simulink model "GalacticSoupLogical"  (R2025b)
settings: Solver=VariableStepAuto  StartTime=0.0  StopTime=10.0  RelTol=1e-3
settings Model: DataDictionary=GalacticSoupLogicalInterfaces.sldd  Creator=sarah  LastModifiedBy=sarah

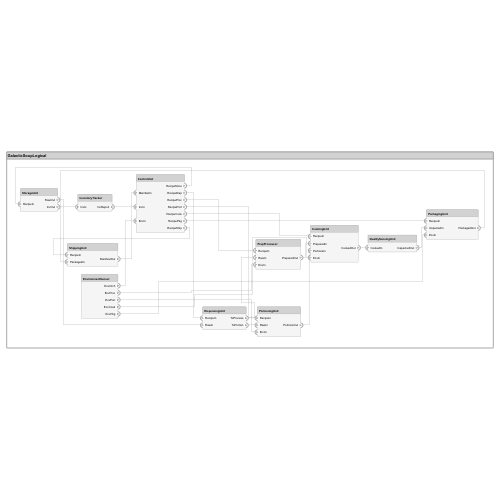
[thumbnail: Simulink's stored preview of the top-level diagram]
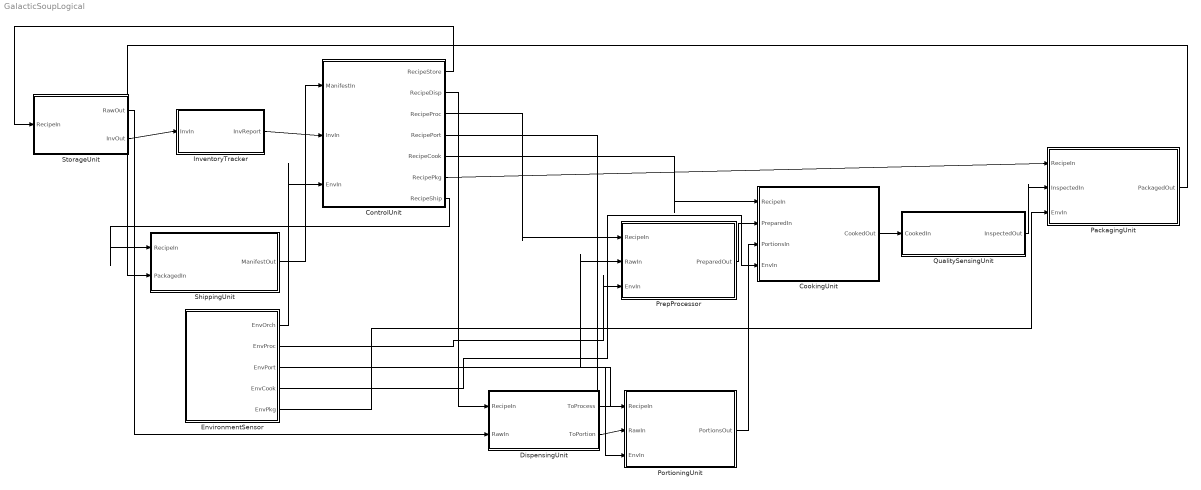
== system GalacticSoupLogical ==
  ControlUnit : Subsystem
      settings: PortSchema="{\"entries\":[{\"content\":{\"headerSize\":26,\"margin\":15,\"minimumSpacing\":25,\"sides\":[{\"content\":{\"connectorIds\":[\"In1\",\"In2\",\"In3\"]},\"type\":\"ConnectorPlacement.EquallySpacedRectSide\",\"uuid\":\"e444b18e-2ceb-4425-8803-e6c31b1fcd82\"},{\"content\":{\"connectorIds\":[\"Out1\",\"Out2\",\"Out3\",\"Out4\",\"Out5\",\"Out6\",\"Out7\"],\"side\":\"RIGHT\"},\"type\":\"ConnectorPlacement.EquallySpacedRectSide\",\"uuid\":\"f4aec6c9-b52d-4884-9c27-2bb07598a416\"},{\"content\":{\"side\":\"TOP\"},\"type\":\"ConnectorPlacement.EquallySpacedRectSide\",\"uuid\":\"1037694d-1bab-41f9-830b-c4a2d0bddcad\"}]},\"type\":\"ConnectorPlacement.EquallySpacedConnector\",\"uuid\":\"fcfa453c-694a-4044-b0a2-73b33e092223\"}],\"packageUris\":[\"http://schema.mathworks.com/mf0/Connector/R2020b\"],\"version\":\"1.0\"}"
  CookingUnit : Subsystem
      settings: PortSchema="{\"entries\":[{\"content\":{\"headerSize\":26,\"margin\":15,\"minimumSpacing\":25,\"sides\":[{\"content\":{\"connectorIds\":[\"In1\",\"In2\",\"In3\",\"In4\"]},\"type\":\"ConnectorPlacement.EquallySpacedRectSide\",\"uuid\":\"e444b18e-2ceb-4425-8803-e6c31b1fcd82\"},{\"content\":{\"connectorIds\":[\"Out1\"],\"side\":\"RIGHT\"},\"type\":\"ConnectorPlacement.EquallySpacedRectSide\",\"uuid\":\"f4aec6c9-b52d-4884-9c27-2bb07598a416\"},{\"content\":{\"side\":\"TOP\"},\"type\":\"ConnectorPlacement.EquallySpacedRectSide\",\"uuid\":\"1037694d-1bab-41f9-830b-c4a2d0bddcad\"}]},\"type\":\"ConnectorPlacement.EquallySpacedConnector\",\"uuid\":\"fcfa453c-694a-4044-b0a2-73b33e092223\"}],\"packageUris\":[\"http://schema.mathworks.com/mf0/Connector/R2020b\"],\"version\":\"1.0\"}"
  DispensingUnit : Subsystem
      settings: PortSchema="{\"entries\":[{\"content\":{\"headerSize\":26,\"margin\":15,\"minimumSpacing\":25,\"sides\":[{\"content\":{\"connectorIds\":[\"In1\",\"In2\"]},\"type\":\"ConnectorPlacement.EquallySpacedRectSide\",\"uuid\":\"e444b18e-2ceb-4425-8803-e6c31b1fcd82\"},{\"content\":{\"connectorIds\":[\"Out1\",\"Out2\"],\"side\":\"RIGHT\"},\"type\":\"ConnectorPlacement.EquallySpacedRectSide\",\"uuid\":\"f4aec6c9-b52d-4884-9c27-2bb07598a416\"},{\"content\":{\"side\":\"TOP\"},\"type\":\"ConnectorPlacement.EquallySpacedRectSide\",\"uuid\":\"1037694d-1bab-41f9-830b-c4a2d0bddcad\"}]},\"type\":\"ConnectorPlacement.EquallySpacedConnector\",\"uuid\":\"fcfa453c-694a-4044-b0a2-73b33e092223\"}],\"packageUris\":[\"http://schema.mathworks.com/mf0/Connector/R2020b\"],\"version\":\"1.0\"}"
  EnvironmentSensor : Subsystem
      settings: PortSchema="{\"entries\":[{\"content\":{\"headerSize\":26,\"margin\":15,\"minimumSpacing\":25,\"sides\":[{\"content\":{},\"type\":\"ConnectorPlacement.EquallySpacedRectSide\",\"uuid\":\"e444b18e-2ceb-4425-8803-e6c31b1fcd82\"},{\"content\":{\"connectorIds\":[\"Out1\",\"Out2\",\"Out3\",\"Out4\",\"Out5\"],\"side\":\"RIGHT\"},\"type\":\"ConnectorPlacement.EquallySpacedRectSide\",\"uuid\":\"f4aec6c9-b52d-4884-9c27-2bb07598a416\"},{\"content\":{\"side\":\"TOP\"},\"type\":\"ConnectorPlacement.EquallySpacedRectSide\",\"uuid\":\"1037694d-1bab-41f9-830b-c4a2d0bddcad\"}]},\"type\":\"ConnectorPlacement.EquallySpacedConnector\",\"uuid\":\"fcfa453c-694a-4044-b0a2-73b33e092223\"}],\"packageUris\":[\"http://schema.mathworks.com/mf0/Connector/R2020b\"],\"version\":\"1.0\"}"
  InventoryTracker : Subsystem
      settings: PortSchema="{\"entries\":[{\"content\":{\"headerSize\":26,\"margin\":15,\"minimumSpacing\":25,\"sides\":[{\"content\":{\"connectorIds\":[\"In1\"]},\"type\":\"ConnectorPlacement.EquallySpacedRectSide\",\"uuid\":\"e444b18e-2ceb-4425-8803-e6c31b1fcd82\"},{\"content\":{\"connectorIds\":[\"Out1\"],\"side\":\"RIGHT\"},\"type\":\"ConnectorPlacement.EquallySpacedRectSide\",\"uuid\":\"f4aec6c9-b52d-4884-9c27-2bb07598a416\"},{\"content\":{\"side\":\"TOP\"},\"type\":\"ConnectorPlacement.EquallySpacedRectSide\",\"uuid\":\"1037694d-1bab-41f9-830b-c4a2d0bddcad\"}]},\"type\":\"ConnectorPlacement.EquallySpacedConnector\",\"uuid\":\"fcfa453c-694a-4044-b0a2-73b33e092223\"}],\"packageUris\":[\"http://schema.mathworks.com/mf0/Connector/R2020b\"],\"version\":\"1.0\"}"
  PackagingUnit : Subsystem
      settings: PortSchema="{\"entries\":[{\"content\":{\"headerSize\":26,\"margin\":15,\"minimumSpacing\":25,\"sides\":[{\"content\":{\"connectorIds\":[\"In1\",\"In2\",\"In3\"]},\"type\":\"ConnectorPlacement.EquallySpacedRectSide\",\"uuid\":\"e444b18e-2ceb-4425-8803-e6c31b1fcd82\"},{\"content\":{\"connectorIds\":[\"Out1\"],\"side\":\"RIGHT\"},\"type\":\"ConnectorPlacement.EquallySpacedRectSide\",\"uuid\":\"f4aec6c9-b52d-4884-9c27-2bb07598a416\"},{\"content\":{\"side\":\"TOP\"},\"type\":\"ConnectorPlacement.EquallySpacedRectSide\",\"uuid\":\"1037694d-1bab-41f9-830b-c4a2d0bddcad\"}]},\"type\":\"ConnectorPlacement.EquallySpacedConnector\",\"uuid\":\"fcfa453c-694a-4044-b0a2-73b33e092223\"}],\"packageUris\":[\"http://schema.mathworks.com/mf0/Connector/R2020b\"],\"version\":\"1.0\"}"
  PortioningUnit : Subsystem
      settings: PortSchema="{\"entries\":[{\"content\":{\"headerSize\":26,\"margin\":15,\"minimumSpacing\":25,\"sides\":[{\"content\":{\"connectorIds\":[\"In1\",\"In2\",\"In3\"]},\"type\":\"ConnectorPlacement.EquallySpacedRectSide\",\"uuid\":\"e444b18e-2ceb-4425-8803-e6c31b1fcd82\"},{\"content\":{\"connectorIds\":[\"Out1\"],\"side\":\"RIGHT\"},\"type\":\"ConnectorPlacement.EquallySpacedRectSide\",\"uuid\":\"f4aec6c9-b52d-4884-9c27-2bb07598a416\"},{\"content\":{\"side\":\"TOP\"},\"type\":\"ConnectorPlacement.EquallySpacedRectSide\",\"uuid\":\"1037694d-1bab-41f9-830b-c4a2d0bddcad\"}]},\"type\":\"ConnectorPlacement.EquallySpacedConnector\",\"uuid\":\"fcfa453c-694a-4044-b0a2-73b33e092223\"}],\"packageUris\":[\"http://schema.mathworks.com/mf0/Connector/R2020b\"],\"version\":\"1.0\"}"
  PrepProcessor : Subsystem
      settings: PortSchema="{\"entries\":[{\"content\":{\"headerSize\":26,\"margin\":15,\"minimumSpacing\":25,\"sides\":[{\"content\":{\"connectorIds\":[\"In1\",\"In2\",\"In3\"]},\"type\":\"ConnectorPlacement.EquallySpacedRectSide\",\"uuid\":\"e444b18e-2ceb-4425-8803-e6c31b1fcd82\"},{\"content\":{\"connectorIds\":[\"Out1\"],\"side\":\"RIGHT\"},\"type\":\"ConnectorPlacement.EquallySpacedRectSide\",\"uuid\":\"f4aec6c9-b52d-4884-9c27-2bb07598a416\"},{\"content\":{\"side\":\"TOP\"},\"type\":\"ConnectorPlacement.EquallySpacedRectSide\",\"uuid\":\"1037694d-1bab-41f9-830b-c4a2d0bddcad\"}]},\"type\":\"ConnectorPlacement.EquallySpacedConnector\",\"uuid\":\"fcfa453c-694a-4044-b0a2-73b33e092223\"}],\"packageUris\":[\"http://schema.mathworks.com/mf0/Connector/R2020b\"],\"version\":\"1.0\"}"
  QualitySensingUnit : Subsystem
      settings: PortSchema="{\"entries\":[{\"content\":{\"headerSize\":26,\"margin\":15,\"minimumSpacing\":25,\"sides\":[{\"content\":{\"connectorIds\":[\"In1\"]},\"type\":\"ConnectorPlacement.EquallySpacedRectSide\",\"uuid\":\"e444b18e-2ceb-4425-8803-e6c31b1fcd82\"},{\"content\":{\"connectorIds\":[\"Out1\"],\"side\":\"RIGHT\"},\"type\":\"ConnectorPlacement.EquallySpacedRectSide\",\"uuid\":\"f4aec6c9-b52d-4884-9c27-2bb07598a416\"},{\"content\":{\"side\":\"TOP\"},\"type\":\"ConnectorPlacement.EquallySpacedRectSide\",\"uuid\":\"1037694d-1bab-41f9-830b-c4a2d0bddcad\"}]},\"type\":\"ConnectorPlacement.EquallySpacedConnector\",\"uuid\":\"fcfa453c-694a-4044-b0a2-73b33e092223\"}],\"packageUris\":[\"http://schema.mathworks.com/mf0/Connector/R2020b\"],\"version\":\"1.0\"}"
  ShippingUnit : Subsystem
      settings: PortSchema="{\"entries\":[{\"content\":{\"headerSize\":26,\"margin\":15,\"minimumSpacing\":25,\"sides\":[{\"content\":{\"connectorIds\":[\"In1\",\"In2\"]},\"type\":\"ConnectorPlacement.EquallySpacedRectSide\",\"uuid\":\"e444b18e-2ceb-4425-8803-e6c31b1fcd82\"},{\"content\":{\"connectorIds\":[\"Out1\"],\"side\":\"RIGHT\"},\"type\":\"ConnectorPlacement.EquallySpacedRectSide\",\"uuid\":\"f4aec6c9-b52d-4884-9c27-2bb07598a416\"},{\"content\":{\"side\":\"TOP\"},\"type\":\"ConnectorPlacement.EquallySpacedRectSide\",\"uuid\":\"1037694d-1bab-41f9-830b-c4a2d0bddcad\"}]},\"type\":\"ConnectorPlacement.EquallySpacedConnector\",\"uuid\":\"fcfa453c-694a-4044-b0a2-73b33e092223\"}],\"packageUris\":[\"http://schema.mathworks.com/mf0/Connector/R2020b\"],\"version\":\"1.0\"}"
  StorageUnit : Subsystem
      settings: PortSchema="{\"entries\":[{\"content\":{\"headerSize\":26,\"margin\":15,\"minimumSpacing\":25,\"sides\":[{\"content\":{\"connectorIds\":[\"In1\"]},\"type\":\"ConnectorPlacement.EquallySpacedRectSide\",\"uuid\":\"e444b18e-2ceb-4425-8803-e6c31b1fcd82\"},{\"content\":{\"connectorIds\":[\"Out1\",\"Out2\"],\"side\":\"RIGHT\"},\"type\":\"ConnectorPlacement.EquallySpacedRectSide\",\"uuid\":\"f4aec6c9-b52d-4884-9c27-2bb07598a416\"},{\"content\":{\"side\":\"TOP\"},\"type\":\"ConnectorPlacement.EquallySpacedRectSide\",\"uuid\":\"1037694d-1bab-41f9-830b-c4a2d0bddcad\"}]},\"type\":\"ConnectorPlacement.EquallySpacedConnector\",\"uuid\":\"fcfa453c-694a-4044-b0a2-73b33e092223\"}],\"packageUris\":[\"http://schema.mathworks.com/mf0/Connector/R2020b\"],\"version\":\"1.0\"}"
  wires:
  ShippingUnit/1(ManifestOut) -> ControlUnit/1(ManifestIn)
  StorageUnit/1(RawOut) -> DispensingUnit/2(RawIn)
  InventoryTracker/1(InvReport) -> ControlUnit/2(InvIn)
  StorageUnit/2(InvOut) -> InventoryTracker/1(InvIn)
  EnvironmentSensor/2(EnvProc) -> PrepProcessor/3(EnvIn)
  EnvironmentSensor/1(EnvOrch) -> ControlUnit/3(EnvIn)
  EnvironmentSensor/4(EnvCook) -> CookingUnit/4(EnvIn)
  EnvironmentSensor/3(EnvPort) -> PortioningUnit/3(EnvIn)
  EnvironmentSensor/5(EnvPkg) -> PackagingUnit/3(EnvIn)
  ControlUnit/1(RecipeStore) -> StorageUnit/1(RecipeIn)
  PrepProcessor/1(PreparedOut) -> CookingUnit/2(PreparedIn)
  ControlUnit/2(RecipeDisp) -> DispensingUnit/1(RecipeIn)
  ControlUnit/3(RecipeProc) -> PrepProcessor/1(RecipeIn)
  ControlUnit/4(RecipePort) -> PortioningUnit/1(RecipeIn)
  ControlUnit/5(RecipeCook) -> CookingUnit/1(RecipeIn)
  ControlUnit/6(RecipePkg) -> PackagingUnit/1(RecipeIn)
  ControlUnit/7(RecipeShip) -> ShippingUnit/1(RecipeIn)
  DispensingUnit/1(ToProcess) -> PrepProcessor/2(RawIn)
  DispensingUnit/2(ToPortion) -> PortioningUnit/2(RawIn)
  PortioningUnit/1(PortionsOut) -> CookingUnit/3(PortionsIn)
  CookingUnit/1(CookedOut) -> QualitySensingUnit/1(CookedIn)
  QualitySensingUnit/1(InspectedOut) -> PackagingUnit/2(InspectedIn)
  PackagingUnit/1(PackagedOut) -> ShippingUnit/2(PackagedIn)

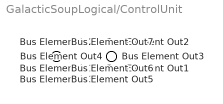
== system GalacticSoupLogical/ControlUnit ==
  Bus Element In1 : Inport  PortName=ManifestIn
  Bus Element In2 : Inport  Port=2  PortName=InvIn
  Bus Element In3 : Inport  Port=3  PortName=EnvIn
  Bus Element Out1 : Outport  PortName=RecipeStore
  Bus Element Out2 : Outport  Port=2  PortName=RecipeDisp
  Bus Element Out3 : Outport  Port=3  PortName=RecipeProc
  Bus Element Out4 : Outport  Port=4  PortName=RecipePort
  Bus Element Out5 : Outport  Port=5  PortName=RecipeCook
  Bus Element Out6 : Outport  Port=6  PortName=RecipePkg
  Bus Element Out7 : Outport  Port=7  PortName=RecipeShip

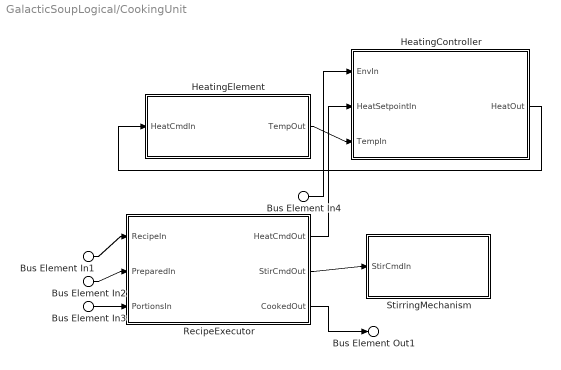
== system GalacticSoupLogical/CookingUnit ==
  Bus Element In1 : Inport  PortName=RecipeIn
  Bus Element In2 : Inport  Port=2  PortName=PreparedIn
  Bus Element In3 : Inport  Port=3  PortName=PortionsIn
  Bus Element In4 : Inport  Port=4  PortName=EnvIn
  HeatingController : Subsystem
      settings: PortSchema="{\"entries\":[{\"content\":{\"headerSize\":26,\"margin\":15,\"minimumSpacing\":25,\"sides\":[{\"content\":{\"connectorIds\":[\"In1\",\"In2\",\"In3\"]},\"type\":\"ConnectorPlacement.EquallySpacedRectSide\",\"uuid\":\"e444b18e-2ceb-4425-8803-e6c31b1fcd82\"},{\"content\":{\"connectorIds\":[\"Out1\"],\"side\":\"RIGHT\"},\"type\":\"ConnectorPlacement.EquallySpacedRectSide\",\"uuid\":\"f4aec6c9-b52d-4884-9c27-2bb07598a416\"},{\"content\":{\"side\":\"TOP\"},\"type\":\"ConnectorPlacement.EquallySpacedRectSide\",\"uuid\":\"1037694d-1bab-41f9-830b-c4a2d0bddcad\"}]},\"type\":\"ConnectorPlacement.EquallySpacedConnector\",\"uuid\":\"fcfa453c-694a-4044-b0a2-73b33e092223\"}],\"packageUris\":[\"http://schema.mathworks.com/mf0/Connector/R2020b\"],\"version\":\"1.0\"}"
  HeatingElement : Subsystem
      settings: PortSchema="{\"entries\":[{\"content\":{\"headerSize\":26,\"margin\":15,\"minimumSpacing\":25,\"sides\":[{\"content\":{\"connectorIds\":[\"In1\"]},\"type\":\"ConnectorPlacement.EquallySpacedRectSide\",\"uuid\":\"e444b18e-2ceb-4425-8803-e6c31b1fcd82\"},{\"content\":{\"connectorIds\":[\"Out1\"],\"side\":\"RIGHT\"},\"type\":\"ConnectorPlacement.EquallySpacedRectSide\",\"uuid\":\"f4aec6c9-b52d-4884-9c27-2bb07598a416\"},{\"content\":{\"side\":\"TOP\"},\"type\":\"ConnectorPlacement.EquallySpacedRectSide\",\"uuid\":\"1037694d-1bab-41f9-830b-c4a2d0bddcad\"}]},\"type\":\"ConnectorPlacement.EquallySpacedConnector\",\"uuid\":\"fcfa453c-694a-4044-b0a2-73b33e092223\"}],\"packageUris\":[\"http://schema.mathworks.com/mf0/Connector/R2020b\"],\"version\":\"1.0\"}"
  RecipeExecutor : Subsystem
      settings: PortSchema="{\"entries\":[{\"content\":{\"headerSize\":26,\"margin\":15,\"minimumSpacing\":25,\"sides\":[{\"content\":{\"connectorIds\":[\"In1\",\"In2\",\"In3\"]},\"type\":\"ConnectorPlacement.EquallySpacedRectSide\",\"uuid\":\"e444b18e-2ceb-4425-8803-e6c31b1fcd82\"},{\"content\":{\"connectorIds\":[\"Out1\",\"Out2\",\"Out3\"],\"side\":\"RIGHT\"},\"type\":\"ConnectorPlacement.EquallySpacedRectSide\",\"uuid\":\"f4aec6c9-b52d-4884-9c27-2bb07598a416\"},{\"content\":{\"side\":\"TOP\"},\"type\":\"ConnectorPlacement.EquallySpacedRectSide\",\"uuid\":\"1037694d-1bab-41f9-830b-c4a2d0bddcad\"}]},\"type\":\"ConnectorPlacement.EquallySpacedConnector\",\"uuid\":\"fcfa453c-694a-4044-b0a2-73b33e092223\"}],\"packageUris\":[\"http://schema.mathworks.com/mf0/Connector/R2020b\"],\"version\":\"1.0\"}"
  StirringMechanism : Subsystem
      settings: PortSchema="{\"entries\":[{\"content\":{\"headerSize\":26,\"margin\":15,\"minimumSpacing\":25,\"sides\":[{\"content\":{\"connectorIds\":[\"In1\"]},\"type\":\"ConnectorPlacement.EquallySpacedRectSide\",\"uuid\":\"e444b18e-2ceb-4425-8803-e6c31b1fcd82\"},{\"content\":{\"side\":\"RIGHT\"},\"type\":\"ConnectorPlacement.EquallySpacedRectSide\",\"uuid\":\"f4aec6c9-b52d-4884-9c27-2bb07598a416\"},{\"content\":{\"side\":\"TOP\"},\"type\":\"ConnectorPlacement.EquallySpacedRectSide\",\"uuid\":\"1037694d-1bab-41f9-830b-c4a2d0bddcad\"}]},\"type\":\"ConnectorPlacement.EquallySpacedConnector\",\"uuid\":\"fcfa453c-694a-4044-b0a2-73b33e092223\"}],\"packageUris\":[\"http://schema.mathworks.com/mf0/Connector/R2020b\"],\"version\":\"1.0\"}"
  Bus Element Out1 : Outport  PortName=CookedOut
  wires:
  Bus Element In1/1 -> RecipeExecutor/1(RecipeIn)
  RecipeExecutor/3(CookedOut) -> Bus Element Out1/1
  Bus Element In2/1 -> RecipeExecutor/2(PreparedIn)
  HeatingElement/1(TempOut) -> HeatingController/3(TempIn)
  Bus Element In3/1 -> RecipeExecutor/3(PortionsIn)
  Bus Element In4/1 -> HeatingController/1(EnvIn)
  RecipeExecutor/1(HeatCmdOut) -> HeatingController/2(HeatSetpointIn)
  RecipeExecutor/2(StirCmdOut) -> StirringMechanism/1(StirCmdIn)
  HeatingController/1(HeatOut) -> HeatingElement/1(HeatCmdIn)

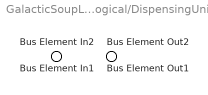
== system GalacticSoupLogical/DispensingUnit ==
  Bus Element In1 : Inport  PortName=RecipeIn
  Bus Element In2 : Inport  Port=2  PortName=RawIn
  Bus Element Out1 : Outport  PortName=ToProcess
  Bus Element Out2 : Outport  Port=2  PortName=ToPortion

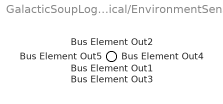
== system GalacticSoupLogical/EnvironmentSensor ==
  Bus Element Out1 : Outport  PortName=EnvOrch
  Bus Element Out2 : Outport  Port=2  PortName=EnvProc
  Bus Element Out3 : Outport  Port=3  PortName=EnvPort
  Bus Element Out4 : Outport  Port=4  PortName=EnvCook
  Bus Element Out5 : Outport  Port=5  PortName=EnvPkg

== system GalacticSoupLogical/InventoryTracker ==
  Bus Element In1 : Inport  PortName=InvIn
  Bus Element Out1 : Outport  PortName=InvReport

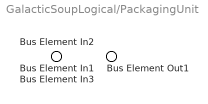
== system GalacticSoupLogical/PackagingUnit ==
  Bus Element In1 : Inport  PortName=RecipeIn
  Bus Element In2 : Inport  Port=2  PortName=InspectedIn
  Bus Element In3 : Inport  Port=3  PortName=EnvIn
  Bus Element Out1 : Outport  PortName=PackagedOut

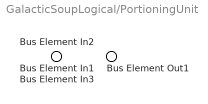
== system GalacticSoupLogical/PortioningUnit ==
  Bus Element In1 : Inport  PortName=RecipeIn
  Bus Element In2 : Inport  Port=2  PortName=RawIn
  Bus Element In3 : Inport  Port=3  PortName=EnvIn
  Bus Element Out1 : Outport  PortName=PortionsOut

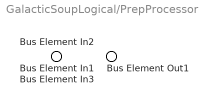
== system GalacticSoupLogical/PrepProcessor ==
  Bus Element In1 : Inport  PortName=RecipeIn
  Bus Element In2 : Inport  Port=2  PortName=RawIn
  Bus Element In3 : Inport  Port=3  PortName=EnvIn
  Bus Element Out1 : Outport  PortName=PreparedOut

== system GalacticSoupLogical/QualitySensingUnit ==
  Bus Element In1 : Inport  PortName=CookedIn
  Bus Element Out1 : Outport  PortName=InspectedOut

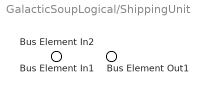
== system GalacticSoupLogical/ShippingUnit ==
  Bus Element In1 : Inport  PortName=RecipeIn
  Bus Element In2 : Inport  Port=2  PortName=PackagedIn
  Bus Element Out1 : Outport  PortName=ManifestOut

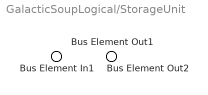
== system GalacticSoupLogical/StorageUnit ==
  Bus Element In1 : Inport  PortName=RecipeIn
  Bus Element Out1 : Outport  PortName=RawOut
  Bus Element Out2 : Outport  Port=2  PortName=InvOut

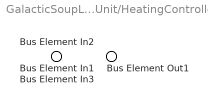
== system GalacticSoupLogical/CookingUnit/HeatingController ==
  Bus Element In1 : Inport  PortName=EnvIn
  Bus Element In2 : Inport  Port=2  PortName=HeatSetpointIn
  Bus Element In3 : Inport  Port=3  PortName=TempIn
  Bus Element Out1 : Outport  PortName=HeatOut

== system GalacticSoupLogical/CookingUnit/HeatingElement ==
  Bus Element In1 : Inport  PortName=HeatCmdIn
  Bus Element Out1 : Outport  PortName=TempOut

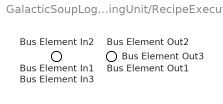
== system GalacticSoupLogical/CookingUnit/RecipeExecutor ==
  Bus Element In1 : Inport  PortName=RecipeIn
  Bus Element In2 : Inport  Port=2  PortName=PreparedIn
  Bus Element In3 : Inport  Port=3  PortName=PortionsIn
  Bus Element Out1 : Outport  PortName=HeatCmdOut
  Bus Element Out2 : Outport  Port=2  PortName=StirCmdOut
  Bus Element Out3 : Outport  Port=3  PortName=CookedOut

== system GalacticSoupLogical/CookingUnit/StirringMechanism ==
  Bus Element In1 : Inport  PortName=StirCmdIn
